simulink model "runningsum"  (R2020b)
settings: Solver=VariableStepAuto  StartTime=0.0  StopTime=10.0  RelTol=1e-3
settings Model: Creator=IIT_KGP_CSE_FM_LAB  LastModifiedBy=IIT_KGP_CSE_FM_LAB

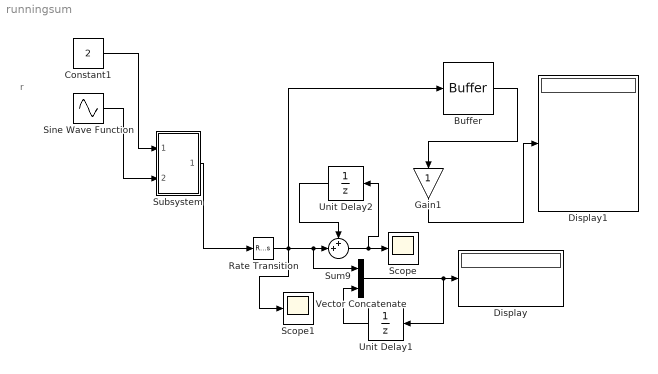
== system runningsum ==
  note: r
  Buffer : Buffer  OutputFrames=off
  Constant1 : Constant  Value=2  SampleTime=-1
  Display : Display
  Display1 : Display
  Gain1 : Gain
  Rate Transition : RateTransition  OutPortSampleTime=1
  Scope : Scope
  Scope1 : Scope
  Sine Wave Function : Sin  Amplitude=4  SampleTime=0
  Subsystem : Subsystem
  Sum9 : Sum  Inputs=++|
  Unit Delay1 : UnitDelay  SampleTime=-1  HasFrameUpgradeWarning=on
  Unit Delay2 : UnitDelay  SampleTime=-1  HasFrameUpgradeWarning=on
  Vector Concatenate : Concatenate  Mode=Multidimensional array
  wires:
  Unit Delay2/1 -> Sum9/1
  Sum9/1 -> Scope/1, Unit Delay2/1
  Rate Transition/1 -> Scope1/1, Buffer/1, Vector Concatenate/1, Sum9/2
  Gain1/1 -> Display1/1
  Vector Concatenate/1 -> Unit Delay1/1, Display/1
  Unit Delay1/1 -> Vector Concatenate/2
  Buffer/1 -> Gain1/1
  Constant1/1 -> Subsystem/1(In1)
  Sine Wave Function/1 -> Subsystem/2(In2)
  Subsystem/1(Out1) -> Rate Transition/1

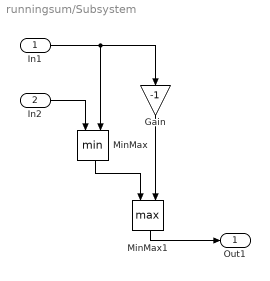
== system runningsum/Subsystem ==
  In1 : Inport
  In2 : Inport  Port=2
  Gain : Gain  Gain=-1
  MinMax : MinMax  Inputs=2
  MinMax1 : MinMax  Function=max  Inputs=2
  Out1 : Outport
  wires:
  In1/1 -> MinMax/2, Gain/1
  Gain/1 -> MinMax1/2
  MinMax/1 -> MinMax1/1
  MinMax1/1 -> Out1/1
  In2/1 -> MinMax/1
